simulink model "CH3_2"  (Simulink 5.0)
settings: Solver=ode15s  SolverMode=SingleTasking  StartTime=0.0  StopTime=3/60  RelTol=1e-3  AbsTol=1e-3
libraries: powerlib2 x10, powerlib_extras x3
Description:
  | 高苑科技大學 電機系
  | 電力電子實驗室
settings Model: Creator=徐瑞隆老師  LastModifiedBy=ELECTRONIC  ExtModeTrigMode=oneshot  ExtModeArmWhenConnect=off  MaxOrder=4  LimitDataPoints=off  BlockReductionOpt=off  BooleanDataType=off  RTWTemplateMakefile=grt_unix.tmf

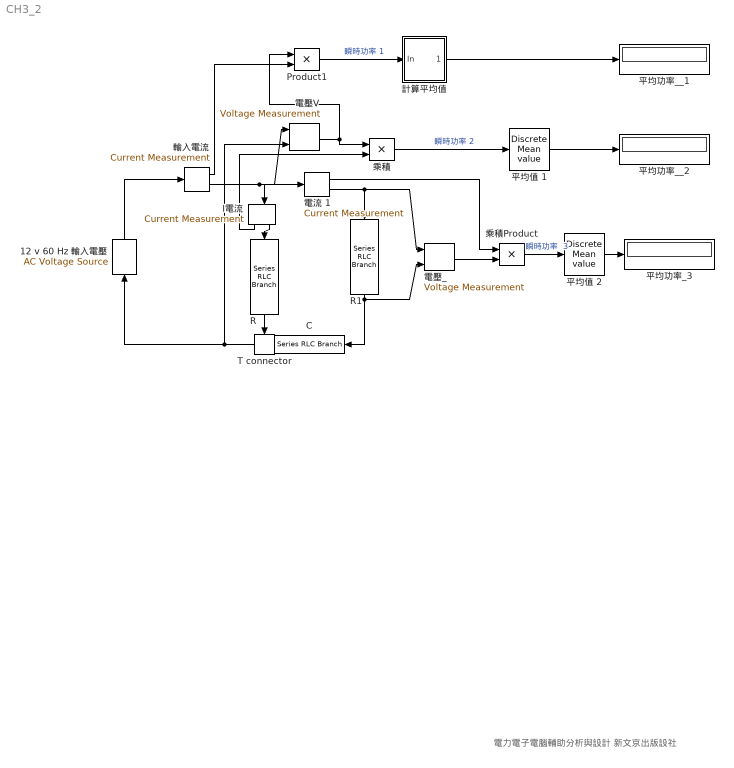
== system CH3_2 ==
  note: 電力電子電腦輔助分析與設計 新文京出版設社
  12 v 60 Hz 輸入電壓 : powerlib2/Electrical Sources/AC Voltage Source  Tag=PoWeRsYsTeMbLoCk  Orientation=up  A=12  P=45  F=60  stime=0  mesure=None  PSBOutputType=1
  C : powerlib2/Elements/Series RLC Branch  Tag=PoWeRsYsTeMbLoCk  Orientation=left  a=0  b=0e-3  c=2600e-6  mesure=None  PSBOutputType=1
  "I電流 " : powerlib2/Measurements/Current Measurement  Tag=PoWeRsYsTeMmEaSuReMeNt  Orientation=down  PhasorSimulation=off  OutputType=Magnitude  PSBOutputType=01  PSBequivalent=0
  Product1 : Product  SaturateOnIntegerOverflow=on
  "R  " : powerlib2/Elements/Series RLC Branch  Tag=PoWeRsYsTeMbLoCk  Orientation=down  a=4  b=0e-3  c=inf  mesure=None  PSBOutputType=1
  R1 : powerlib2/Elements/Series RLC Branch  Tag=PoWeRsYsTeMbLoCk  Orientation=down  a=2  b=0e-3  c=inf  mesure=None  PSBOutputType=1
  T connector : powerlib2/Connectors/T connector  Tag=PoWeRsYsTeMbLoCk  Orientation=left  PSBOutputType=1
  平均功率_3 : Display
  平均功率__1 : Display
  平均功率__2 : Display
  平均值 1 : powerlib_extras/Discrete Measurements/Discrete  Mean value  AncestorBlock=|  Freq=60  Vinit=0  Ts=50e-6
      | powerlib_extras/Discrete
      | Measurements/Discrete 
      | Mean value
  平均值 2 : powerlib_extras/Discrete Measurements/Discrete  Mean value  AncestorBlock=|  Freq=60  Vinit=0  Ts=50e-6
      | powerlib_extras/Discrete
      | Measurements/Discrete 
      | Mean value
  "計算平均值 " : Subsystem  AncestorBlock=|  mask(Discrete Mean value){Freq=60, Vinit=0, Ts=50e-6}
      | powerlib_extras/Discrete
      | Measurements/Discrete 
      | Mean value
      mask prompts: Freq "Fundamental frequency (Hz):"; Vinit "Initial input (DC component):"; Ts "Sample time:"
      mask help:
      | This block computes the mean value of the input signal over a running window of one cycle of the specified fundamental frequency.
      | For the first cycle of simulation, the ouput is held constant to the value specified by the parameter "Initial input".
      mask init:
      | SamplesPerCycle=1/Freq/Ts;
      | RoundSamplesPerCycle=ceil(SamplesPerCycle);
      | Delay=RoundSamplesPerCycle*Ts;
      | Corr1=(SamplesPerCycle-RoundSamplesPerCycle)/2;
      | Corr2=(SamplesPerCycle-RoundSamplesPerCycle)/SamplesPerCycle;
      | K1=Corr1*Corr2;
      | K2=Corr2 + Corr1*Corr2;
  乘積 : Product  SaturateOnIntegerOverflow=on
  乘積Product : Product  SaturateOnIntegerOverflow=on
  電流 1 : powerlib2/Measurements/Current Measurement  Tag=PoWeRsYsTeMmEaSuReMeNt  PhasorSimulation=off  OutputType=Magnitude  PSBOutputType=01  PSBequivalent=0
  電壓V : powerlib2/Measurements/Voltage Measurement  Tag=PoWeRsYsTeMmEaSuReMeNt  PhasorSimulation=off  OutputType=Magnitude  PSBOutputType=0  PSBequivalent=0
  電壓_ : powerlib2/Measurements/Voltage Measurement  Tag=PoWeRsYsTeMmEaSuReMeNt  PhasorSimulation=off  OutputType=Magnitude  PSBOutputType=0  PSBequivalent=0
  輸入電流 : powerlib2/Measurements/Current Measurement  Tag=PoWeRsYsTeMmEaSuReMeNt  PhasorSimulation=off  OutputType=Magnitude  PSBOutputType=01  PSBequivalent=0
  wires:
  "計算平均值 "/1(Mean) -> 平均功率__1/1
  12 v 60 Hz 輸入電壓/1 -> 輸入電流/1
  輸入電流/2 -> "I電流 "/1, 電流 1/1, 電壓V/1
  "I電流 "/2 -> "R  "/1
  電流 1/2 -> R1/1, 電壓_/1
  T connector/1 -> 12 v 60 Hz 輸入電壓/1, 電壓V/2
  C/1 -> T connector/1
  輸入電流/1 -> Product1/2
  Product1/1 -> "計算平均值 "/1(In)  "瞬時功率 1"
  電壓V/1 -> 乘積/1, Product1/1
  "I電流 "/1 -> 乘積/2
  電壓_/1 -> 乘積Product/2
  電流 1/1 -> 乘積Product/1
  乘積/1 -> 平均值 1/1  "瞬時功率 2"
  平均值 1/1 -> 平均功率__2/1
  乘積Product/1 -> 平均值 2/1  "瞬時功率  3"
  平均值 2/1 -> 平均功率_3/1
  "R  "/1 -> T connector/Enable
  R1/1 -> C/1, 電壓_/2

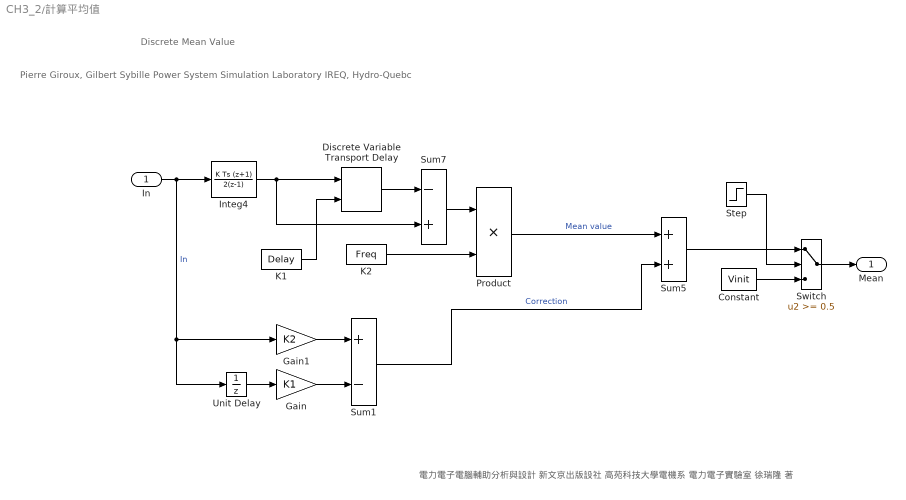
== system CH3_2/計算平均值  ==
  note: Pierre Giroux, Gilbert Sybille
      | Power System Simulation Laboratory
      | IREQ, Hydro-Quebc
  note: Discrete Mean Value
  note: 電力電子電腦輔助分析與設計  新文京出版設社
      | 高苑科技大學電機系
      | 電力電子實驗室
      | 徐瑞隆 著
  In : Inport
  Constant : Constant  Value=Vinit
  Discrete Variable Transport Delay : powerlib_extras/Discrete  Control Blocks/Discrete Variable Transport Delay  MaxDelay=Delay+Ts  InitialValue=0  Ts=Ts
  Gain : Gain  Gain=K1  SaturateOnIntegerOverflow=on
  Gain1 : Gain  Gain=K2  SaturateOnIntegerOverflow=on
  Integ4 : DiscreteIntegrator  IntegratorMethod=Trapezoidal  SampleTime=Ts
  K1 : Constant  Value=Delay
  K2 : Constant  Value=Freq
  Product : Product  SaturateOnIntegerOverflow=on  InputSameDT=on
  Step : Step  Time=1/Freq  SampleTime=Ts
  Sum1 : Sum  Inputs=+-  SaturateOnIntegerOverflow=on  InputSameDT=on
  Sum5 : Sum  SaturateOnIntegerOverflow=on  InputSameDT=on
  Sum7 : Sum  Inputs=-+  SaturateOnIntegerOverflow=on  InputSameDT=on
  Switch : Switch  Threshold=0.5  InputSameDT=on
  Unit Delay : UnitDelay  SampleTime=Ts
  Mean : Outport
  wires:
  Product/1 -> Sum5/1  "Mean value"
  Sum7/1 -> Product/1
  Integ4/1 -> Discrete Variable Transport Delay/1, Sum7/2
  K2/1 -> Product/2
  In/1 -> Integ4/1, Gain1/1, Unit Delay/1  "In"
  Sum5/1 -> Switch/1
  Step/1 -> Switch/2
  Constant/1 -> Switch/3
  Switch/1 -> Mean/1
  Discrete Variable Transport Delay/1 -> Sum7/1
  K1/1 -> Discrete Variable Transport Delay/2
  Gain1/1 -> Sum1/1
  Unit Delay/1 -> Gain/1
  Gain/1 -> Sum1/2
  Sum1/1 -> Sum5/2  "Correction"
